simulink model "CombinedTractionLaunchControl"  (R2019b)
settings: Solver=ode1  StartTime=0.0  StopTime=inf  FixedStep=0.0002  RelTol=1e-3
PreLoadFcn:
  | vehicle = 'Car'; if ~length(which('cmself')), cmenv; end
  | CombinedTractionLaunchControl_bus
InitFcn:
  | vehicle = 'Car'; if ~length(which('cmself')), cmenv; end
  | CombinedTractionLaunchControl_bus
libraries: CarMaker4SL x32
(part 2 of 2)

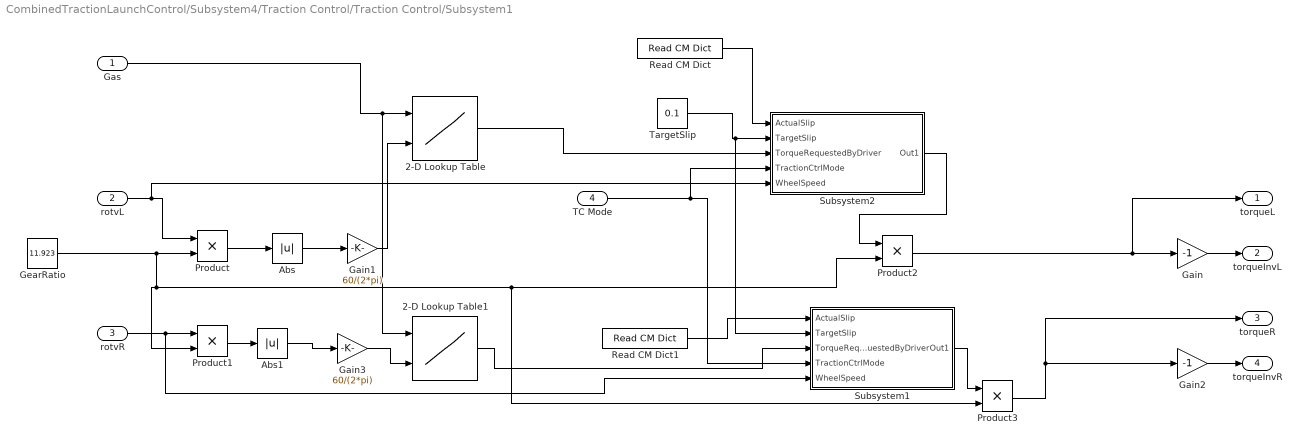
== system CombinedTractionLaunchControl/Subsystem4/Traction Control/Traction Control/Subsystem1 ==
  Gas : Inport
  rotvL : Inport  Port=2
  rotvR : Inport  Port=3
  TC Mode : Inport  Port=4
  2-D Lookup Table : Lookup_n-D  BreakpointsForDimension1=[0 0.2 0.4 0.6 0.8 1]  BreakpointsForDimension2=[0 2000 4000 6000 8000 10000 12000 14000 15000 16000 17000 18000 20000 22000]  Table=[0 0 0 0 0 0 0 0 0 0 0 0 0 0;4 4 4 4 4 4 4 4 4 4 4 4 3 0;8 8 8 8 8 8 8 8 8 8 8 8 6 0;13 13 13 13 13 13 13 13 13 12 12 11 9 0;17 17 17 17 17 17 17 17 17 16 16 15 12 0;21 21 21 21 21 21 21 21 21 20 20 19 15 0]  InternalRulePriority=Speed  RndMeth=Simplest  InputSameDT=on
  2-D Lookup Table1 : Lookup_n-D  BreakpointsForDimension1=[0 0.2 0.4 0.6 0.8 1]  BreakpointsForDimension2=[0 2000 4000 6000 8000 10000 12000 14000 15000 16000 17000 18000 20000 22000]  Table=[0 0 0 0 0 0 0 0 0 0 0 0 0 0;4 4 4 4 4 4 4 4 4 4 4 4 3 0;8 8 8 8 8 8 8 8 8 8 8 8 6 0;13 13 13 13 13 13 13 13 13 12 12 11 9 0;17 17 17 17 17 17 17 17 17 16 16 15 12 0;21 21 21 21 21 21 21 21 21 20 20 19 15 0]  InternalRulePriority=Speed  RndMeth=Simplest  InputSameDT=on
  Abs : Abs
  Abs1 : Abs
  Gain : Gain  Gain=-1
  Gain1 : Gain  Gain=60/(2*pi)
  Gain2 : Gain  Gain=-1
  Gain3 : Gain  Gain=60/(2*pi)
  GearRatio : Constant  Value=11.923
  Product{,1..3} (4 alike) : Product
  Read CM Dict : CarMaker4SL/Read CM Dict  xname=Car.LongSlipFL  xsync=off
  Read CM Dict1 : CarMaker4SL/Read CM Dict  xname=Car.LongSlipFR  xsync=off
  Subsystem1 : Subsystem
  Subsystem2 : Subsystem
  TargetSlip : Constant  Value=0.1
  torqueL : Outport
  torqueInvL : Outport  Port=2
  torqueR : Outport  Port=3
  torqueInvR : Outport  Port=4
  wires:
  Gain/1 -> torqueInvL/1
  Product/1 -> Abs/1
  Gas/1 -> 2-D Lookup Table1/1, 2-D Lookup Table/1
  GearRatio/1 -> Product1/2, Product2/2, Product3/2, Product/2
  rotvL/1 -> Subsystem2/5(WheelSpeed), Product/1
  Product2/1 -> Gain/1, torqueL/1
  Abs/1 -> Gain1/1
  Gain1/1 -> 2-D Lookup Table/2
  Gain2/1 -> torqueInvR/1
  rotvR/1 -> Subsystem1/5(WheelSpeed), Product1/1
  Gain3/1 -> 2-D Lookup Table1/2
  Product1/1 -> Abs1/1
  Abs1/1 -> Gain3/1
  Product3/1 -> torqueR/1, Gain2/1
  Subsystem2/1(Out1) -> Product2/1
  Subsystem1/1(Out1) -> Product3/1
  2-D Lookup Table1/1 -> Subsystem1/3(TorqueRequestedByDriver)
  2-D Lookup Table/1 -> Subsystem2/3(TorqueRequestedByDriver)
  TC Mode/1 -> Subsystem1/4(TractionCtrlMode), Subsystem2/4(TractionCtrlMode)
  TargetSlip/1 -> Subsystem1/2(TargetSlip), Subsystem2/2(TargetSlip)
  Read CM Dict1/1 -> Subsystem1/1(ActualSlip)
  Read CM Dict/1 -> Subsystem2/1(ActualSlip)

== system CombinedTractionLaunchControl/Subsystem4/Launch Control/LaunchControl/Subsystem/If Action Subsystem ==
  In1 : Inport
  Action Port : ActionPort  ActionPortLabel=if(u2< u1)
  Out1 : Outport
  wires:
  In1/1 -> Out1/1

== system CombinedTractionLaunchControl/Subsystem4/Launch Control/LaunchControl/Subsystem/If Action Subsystem1 ==
  In1 : Inport
  Action Port : ActionPort  ActionPortLabel=else
  Out1 : Outport
  wires:
  In1/1 -> Out1/1

== system CombinedTractionLaunchControl/Subsystem4/Launch Control/LaunchControl/Subsystem1/If Action Subsystem ==
  In1 : Inport
  Action Port : ActionPort  ActionPortLabel=if(u2< u1)
  Out1 : Outport
  wires:
  In1/1 -> Out1/1

== system CombinedTractionLaunchControl/Subsystem4/Launch Control/LaunchControl/Subsystem1/If Action Subsystem1 ==
  In1 : Inport
  Action Port : ActionPort  ActionPortLabel=else
  Out1 : Outport
  wires:
  In1/1 -> Out1/1

== system CombinedTractionLaunchControl/Subsystem4/Launch Control/LaunchControl/Subsystem2/If Action Subsystem ==
  In1 : Inport
  Action Port : ActionPort  ActionPortLabel=if(u2< u1)
  Out1 : Outport
  wires:
  In1/1 -> Out1/1

== system CombinedTractionLaunchControl/Subsystem4/Launch Control/LaunchControl/Subsystem2/If Action Subsystem1 ==
  In1 : Inport
  Action Port : ActionPort  ActionPortLabel=else
  Out1 : Outport
  wires:
  In1/1 -> Out1/1

== system CombinedTractionLaunchControl/Subsystem4/Launch Control/LaunchControl/Subsystem3/If Action Subsystem ==
  In1 : Inport
  Action Port : ActionPort  ActionPortLabel=if(u2< u1)
  Out1 : Outport
  wires:
  In1/1 -> Out1/1

== system CombinedTractionLaunchControl/Subsystem4/Launch Control/LaunchControl/Subsystem3/If Action Subsystem1 ==
  In1 : Inport
  Action Port : ActionPort  ActionPortLabel=else
  Out1 : Outport
  wires:
  In1/1 -> Out1/1

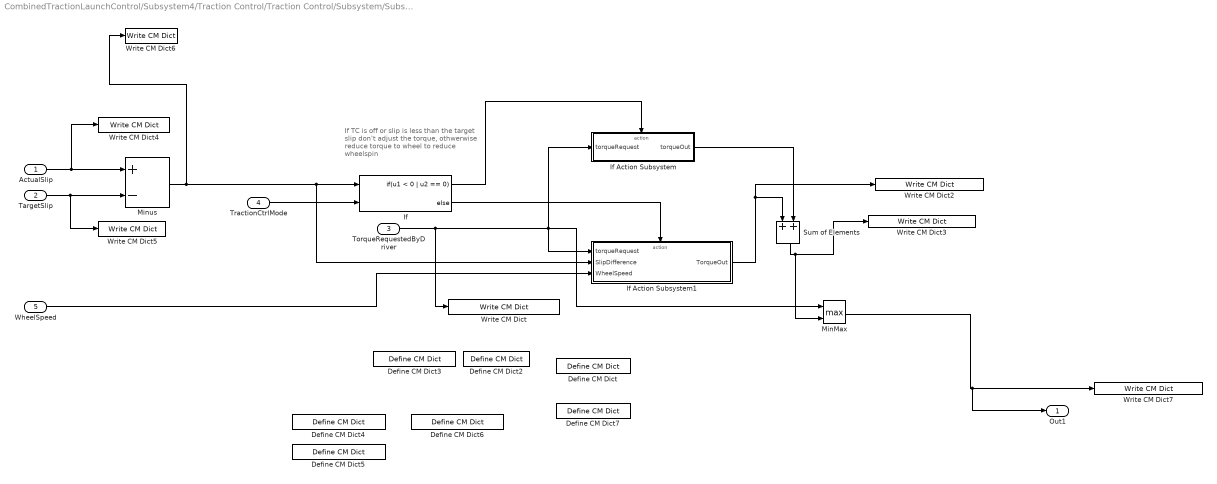
== system CombinedTractionLaunchControl/Subsystem4/Traction Control/Traction Control/Subsystem/Subsystem ==
  note: If TC is off or slip is less than the target slip don't adjust the torque,
      | othwerwise reduce torque to wheel to reduce wheelspin
  ActualSlip : Inport
  TargetSlip : Inport  Port=2
  TorqueRequestedByDriver : Inport  Port=3
  TractionCtrlMode : Inport  Port=4
  WheelSpeed : Inport  Port=5
  Define CM Dict : CarMaker4SL/Define CM Dict  xname=Caleb.TorquePidOut  xmono=off  xtype=Double4  xdvaplace=None  xnstates=0  xfirststate=0  xinitial=0
  Define CM Dict2 : CarMaker4SL/Define CM Dict  xname=Caleb.IfOutput  xmono=off  xtype=Double4  xdvaplace=None  xnstates=0  xfirststate=0  xinitial=0
  Define CM Dict3 : CarMaker4SL/Define CM Dict  xname=Caleb.TorqueRequest  xmono=off  xtype=Double4  xdvaplace=None  xnstates=0  xfirststate=0  xinitial=0
  Define CM Dict4 : CarMaker4SL/Define CM Dict  xname=Caleb.TargetSlip  xmono=off  xtype=Double4  xdvaplace=None  xnstates=0  xfirststate=0  xinitial=0
  Define CM Dict5 : CarMaker4SL/Define CM Dict  xname=Caleb.ActualSlip  xmono=off  xtype=Double4  xdvaplace=None  xnstates=0  xfirststate=0  xinitial=0
  Define CM Dict6 : CarMaker4SL/Define CM Dict  xname=Caleb.DiffSlip  xmono=off  xtype=Double4  xdvaplace=None  xnstates=0  xfirststate=0  xinitial=0
  Define CM Dict7 : CarMaker4SL/Define CM Dict  xname=Caleb.TorqueOut  xmono=off  xtype=Double4  xdvaplace=None  xnstates=0  xfirststate=0  xinitial=0
  If : If  NumInputs=2  IfExpression=u1 < 0 | u2 == 0
  If Action Subsystem : Subsystem  TreatAsAtomicUnit=on
  If Action Subsystem1 : Subsystem  TreatAsAtomicUnit=on
  MinMax : MinMax  Function=max  Inputs=2
  Minus : Sum  Inputs=+-
  Sum of Elements : Sum  Inputs=2
  Write CM Dict : CarMaker4SL/Write CM Dict  xname=Caleb.TorqueRequest  xsync=off
  Write CM Dict2 : CarMaker4SL/Write CM Dict  xname=Caleb.IfOutput  xsync=off
  Write CM Dict3 : CarMaker4SL/Write CM Dict  xname=Caleb.TorquePidOut  xsync=off
  Write CM Dict4 : CarMaker4SL/Write CM Dict  xname=Caleb.TargetSlip  xsync=off
  Write CM Dict5 : CarMaker4SL/Write CM Dict  xname=Caleb.ActualSlip  xsync=off
  Write CM Dict6 : CarMaker4SL/Write CM Dict  xname=Caleb.DiffSlip  xsync=off
  Write CM Dict7 : CarMaker4SL/Write CM Dict  xname=Caleb.TorqueOut  xsync=off
  Out1 : Outport
  wires:
  If Action Subsystem1/1(TorqueOut) -> Write CM Dict2/1, Sum of Elements/1
  TorqueRequestedByDriver/1 -> Write CM Dict/1, If Action Subsystem1/1(torqueRequest), MinMax/1, If Action Subsystem/1(torqueRequest)
  If/1 -> If Action Subsystem/Action
  If Action Subsystem/1(torqueOut) -> Sum of Elements/2
  ActualSlip/1 -> Write CM Dict4/1, Minus/1
  Minus/1 -> Write CM Dict6/1, If Action Subsystem1/2(SlipDifference), If/1
  Sum of Elements/1 -> MinMax/2, Write CM Dict3/1
  TargetSlip/1 -> Write CM Dict5/1, Minus/2
  If/2 -> If Action Subsystem1/Action
  TractionCtrlMode/1 -> If/2
  MinMax/1 -> Out1/1, Write CM Dict7/1
  WheelSpeed/1 -> If Action Subsystem1/3(WheelSpeed)

== system CombinedTractionLaunchControl/Subsystem4/Traction Control/Traction Control/Subsystem/Subsystem1 ==
  note: If TC is off or slip is less than the target slip don't adjust the torque,
      | othwerwise reduce torque to wheel to reduce wheelspin
  ActualSlip : Inport
  TargetSlip : Inport  Port=2
  TorqueRequestedByDriver : Inport  Port=3
  TractionCtrlMode : Inport  Port=4
  WheelSpeed : Inport  Port=5
  If : If  NumInputs=2  IfExpression=u1 < 0 | u2 == 0
  If Action Subsystem : Subsystem  TreatAsAtomicUnit=on
  If Action Subsystem1 : Subsystem  TreatAsAtomicUnit=on
  MinMax : MinMax  Function=max  Inputs=2
  Minus : Sum  Inputs=+-
  Sum of Elements : Sum  Inputs=2
  Out1 : Outport
  wires:
  If Action Subsystem1/1(TorqueOut) -> Sum of Elements/1
  TorqueRequestedByDriver/1 -> If Action Subsystem1/1(torqueRequest), MinMax/1, If Action Subsystem/1(torqueRequest)
  If/1 -> If Action Subsystem/Action
  If Action Subsystem/1(torqueOut) -> Sum of Elements/2
  ActualSlip/1 -> Minus/1
  Minus/1 -> If Action Subsystem1/2(SlipDifference), If/1
  Sum of Elements/1 -> MinMax/2
  TargetSlip/1 -> Minus/2
  If/2 -> If Action Subsystem1/Action
  TractionCtrlMode/1 -> If/2
  MinMax/1 -> Out1/1
  WheelSpeed/1 -> If Action Subsystem1/3(WheelSpeed)

== system CombinedTractionLaunchControl/Subsystem4/Traction Control/Traction Control/Subsystem1/Subsystem1 ==
  note: If TC is off or slip is less than the target slip don't adjust the torque,
      | othwerwise reduce torque to wheel to reduce wheelspin
  ActualSlip : Inport
  TargetSlip : Inport  Port=2
  TorqueRequestedByDriver : Inport  Port=3
  TractionCtrlMode : Inport  Port=4
  WheelSpeed : Inport  Port=5
  If : If  NumInputs=2  IfExpression=u1 < 0 | u2 == 0
  If Action Subsystem : Subsystem  TreatAsAtomicUnit=on
  If Action Subsystem1 : Subsystem  TreatAsAtomicUnit=on
  MinMax : MinMax  Function=max  Inputs=2
  Minus : Sum  Inputs=+-
  Sum of Elements : Sum  Inputs=2
  Out1 : Outport
  wires:
  If Action Subsystem1/1(TorqueOut) -> Sum of Elements/1
  TorqueRequestedByDriver/1 -> If Action Subsystem1/1(torqueRequest), MinMax/1, If Action Subsystem/1(torqueRequest)
  If/1 -> If Action Subsystem/Action
  If Action Subsystem/1(torqueOut) -> Sum of Elements/2
  ActualSlip/1 -> Minus/1
  Minus/1 -> If Action Subsystem1/2(SlipDifference), If/1
  Sum of Elements/1 -> MinMax/2
  TargetSlip/1 -> Minus/2
  If/2 -> If Action Subsystem1/Action
  TractionCtrlMode/1 -> If/2
  MinMax/1 -> Out1/1
  WheelSpeed/1 -> If Action Subsystem1/3(WheelSpeed)

== system CombinedTractionLaunchControl/Subsystem4/Traction Control/Traction Control/Subsystem1/Subsystem2 ==
  note: If TC is off or slip is less than the target slip don't adjust the torque,
      | othwerwise reduce torque to wheel to reduce wheelspin
  ActualSlip : Inport
  TargetSlip : Inport  Port=2
  TorqueRequestedByDriver : Inport  Port=3
  TractionCtrlMode : Inport  Port=4
  WheelSpeed : Inport  Port=5
  If : If  NumInputs=2  IfExpression=u1 < 0 | u2 == 0
  If Action Subsystem : Subsystem  TreatAsAtomicUnit=on
  If Action Subsystem1 : Subsystem  TreatAsAtomicUnit=on
  MinMax : MinMax  Function=max  Inputs=2
  Minus : Sum  Inputs=+-
  Sum of Elements : Sum  Inputs=2
  Out1 : Outport
  wires:
  If Action Subsystem1/1(TorqueOut) -> Sum of Elements/1
  TorqueRequestedByDriver/1 -> MinMax/1, If Action Subsystem1/1(torqueRequest), If Action Subsystem/1(torqueRequest)
  If/1 -> If Action Subsystem/Action
  If Action Subsystem/1(torqueOut) -> Sum of Elements/2
  ActualSlip/1 -> Minus/1
  Minus/1 -> If Action Subsystem1/2(SlipDifference), If/1
  Sum of Elements/1 -> MinMax/2
  TargetSlip/1 -> Minus/2
  If/2 -> If Action Subsystem1/Action
  TractionCtrlMode/1 -> If/2
  MinMax/1 -> Out1/1
  WheelSpeed/1 -> If Action Subsystem1/3(WheelSpeed)

== system CombinedTractionLaunchControl/Subsystem4/Traction Control/Traction Control/Subsystem/Subsystem/If Action Subsystem ==
  torqueRequest : Inport
  Action Port : ActionPort  ActionPortLabel=if(u1 < 0 | u2 == 0)
  torqueOut : Outport
  wires:
  torqueRequest/1 -> torqueOut/1

== system CombinedTractionLaunchControl/Subsystem4/Traction Control/Traction Control/Subsystem/Subsystem/If Action Subsystem1 ==
  torqueRequest : Inport
  SlipDifference : Inport  Port=2
  WheelSpeed : Inport  Port=3
  Action Port : ActionPort  ActionPortLabel=else
  2-D Lookup Table : Lookup_n-D  BreakpointsForDimension1=[0 0.05 0.1 0.15 0.5 2.5]  BreakpointsForDimension2=[0 500 1000 1500 2000]  Table=[0 0 0 0 0;2 2 2 2 2; 5 5 5 5 5; 7 7 7 7 7; 12 12 12 12 12; 50 50 50 50 50]  InternalRulePriority=Speed  RndMeth=Simplest  InputSameDT=on
  Constant : Constant
  Gain : Gain  Gain=1/100
  If : If  IfExpression=u1 > 1
  If Action Subsystem : Subsystem  TreatAsAtomicUnit=on
  If Action Subsystem1 : Subsystem  TreatAsAtomicUnit=on
  Mult : Product  Inputs=**
  Subtract : Sum  Inputs=+-
  Subtract1 : Sum
  TorqueOut : Outport
  wires:
  torqueRequest/1 -> Mult/1
  Mult/1 -> TorqueOut/1
  SlipDifference/1 -> 2-D Lookup Table/1
  WheelSpeed/1 -> 2-D Lookup Table/2
  Constant/1 -> If Action Subsystem/1(torqueRequest), Subtract/1
  Subtract/1 -> Mult/2
  If/2 -> If Action Subsystem1/Action
  If/1 -> If Action Subsystem/Action
  If Action Subsystem/1(torqueOut) -> Subtract1/1
  If Action Subsystem1/1(torqueOut) -> Subtract1/2
  Subtract1/1 -> Subtract/2
  Gain/1 -> If/1, If Action Subsystem1/1(torqueRequest)
  2-D Lookup Table/1 -> Gain/1

== system CombinedTractionLaunchControl/Subsystem4/Traction Control/Traction Control/Subsystem/Subsystem1/If Action Subsystem ==
  torqueRequest : Inport
  Action Port : ActionPort  ActionPortLabel=if(u1 < 0 | u2 == 0)
  torqueOut : Outport
  wires:
  torqueRequest/1 -> torqueOut/1

== system CombinedTractionLaunchControl/Subsystem4/Traction Control/Traction Control/Subsystem/Subsystem1/If Action Subsystem1 ==
  torqueRequest : Inport
  SlipDifference : Inport  Port=2
  WheelSpeed : Inport  Port=3
  Action Port : ActionPort  ActionPortLabel=else
  2-D Lookup Table : Lookup_n-D  BreakpointsForDimension1=[0 0.05 0.1 0.15 0.5 2.5]  BreakpointsForDimension2=[0 500 1000 1500 2000]  Table=[0 0 0 0 0;2 2 2 2 2; 5 5 5 5 5; 7 7 7 7 7; 12 12 12 12 12; 50 50 50 50 50]  InternalRulePriority=Speed  RndMeth=Simplest  InputSameDT=on
  Constant : Constant
  Gain : Gain  Gain=1/100
  If : If  IfExpression=u1 > 1
  If Action Subsystem : Subsystem  TreatAsAtomicUnit=on
  If Action Subsystem1 : Subsystem  TreatAsAtomicUnit=on
  Mult : Product  Inputs=**
  Subtract : Sum  Inputs=+-
  Subtract1 : Sum
  TorqueOut : Outport
  wires:
  torqueRequest/1 -> Mult/1
  Mult/1 -> TorqueOut/1
  SlipDifference/1 -> 2-D Lookup Table/1
  WheelSpeed/1 -> 2-D Lookup Table/2
  Constant/1 -> If Action Subsystem/1(torqueRequest), Subtract/1
  Subtract/1 -> Mult/2
  If/2 -> If Action Subsystem1/Action
  If/1 -> If Action Subsystem/Action
  If Action Subsystem/1(torqueOut) -> Subtract1/1
  If Action Subsystem1/1(torqueOut) -> Subtract1/2
  Subtract1/1 -> Subtract/2
  Gain/1 -> If/1, If Action Subsystem1/1(torqueRequest)
  2-D Lookup Table/1 -> Gain/1

== system CombinedTractionLaunchControl/Subsystem4/Traction Control/Traction Control/Subsystem1/Subsystem1/If Action Subsystem ==
  torqueRequest : Inport
  Action Port : ActionPort  ActionPortLabel=if(u1 < 0 | u2 == 0)
  torqueOut : Outport
  wires:
  torqueRequest/1 -> torqueOut/1

== system CombinedTractionLaunchControl/Subsystem4/Traction Control/Traction Control/Subsystem1/Subsystem1/If Action Subsystem1 ==
  torqueRequest : Inport
  SlipDifference : Inport  Port=2
  WheelSpeed : Inport  Port=3
  Action Port : ActionPort  ActionPortLabel=else
  2-D Lookup Table : Lookup_n-D  BreakpointsForDimension1=[0 0.05 0.1 0.15 0.5 2.5]  BreakpointsForDimension2=[0 500 1000 1500 2000]  Table=[0 0 0 0 0;2 2 2 2 2; 5 5 5 5 5; 7 7 7 7 7; 12 12 12 12 12; 50 50 50 50 50]  InternalRulePriority=Speed  RndMeth=Simplest  InputSameDT=on
  Constant : Constant
  Gain : Gain  Gain=1/100
  If : If  IfExpression=u1 > 1
  If Action Subsystem : Subsystem  TreatAsAtomicUnit=on
  If Action Subsystem1 : Subsystem  TreatAsAtomicUnit=on
  Mult : Product  Inputs=**
  Subtract : Sum  Inputs=+-
  Subtract1 : Sum
  TorqueOut : Outport
  wires:
  torqueRequest/1 -> Mult/1
  Mult/1 -> TorqueOut/1
  SlipDifference/1 -> 2-D Lookup Table/1
  WheelSpeed/1 -> 2-D Lookup Table/2
  Constant/1 -> If Action Subsystem/1(torqueRequest), Subtract/1
  Subtract/1 -> Mult/2
  If/2 -> If Action Subsystem1/Action
  If/1 -> If Action Subsystem/Action
  If Action Subsystem/1(torqueOut) -> Subtract1/1
  If Action Subsystem1/1(torqueOut) -> Subtract1/2
  Subtract1/1 -> Subtract/2
  Gain/1 -> If/1, If Action Subsystem1/1(torqueRequest)
  2-D Lookup Table/1 -> Gain/1

== system CombinedTractionLaunchControl/Subsystem4/Traction Control/Traction Control/Subsystem1/Subsystem2/If Action Subsystem ==
  torqueRequest : Inport
  Action Port : ActionPort  ActionPortLabel=if(u1 < 0 | u2 == 0)
  torqueOut : Outport
  wires:
  torqueRequest/1 -> torqueOut/1

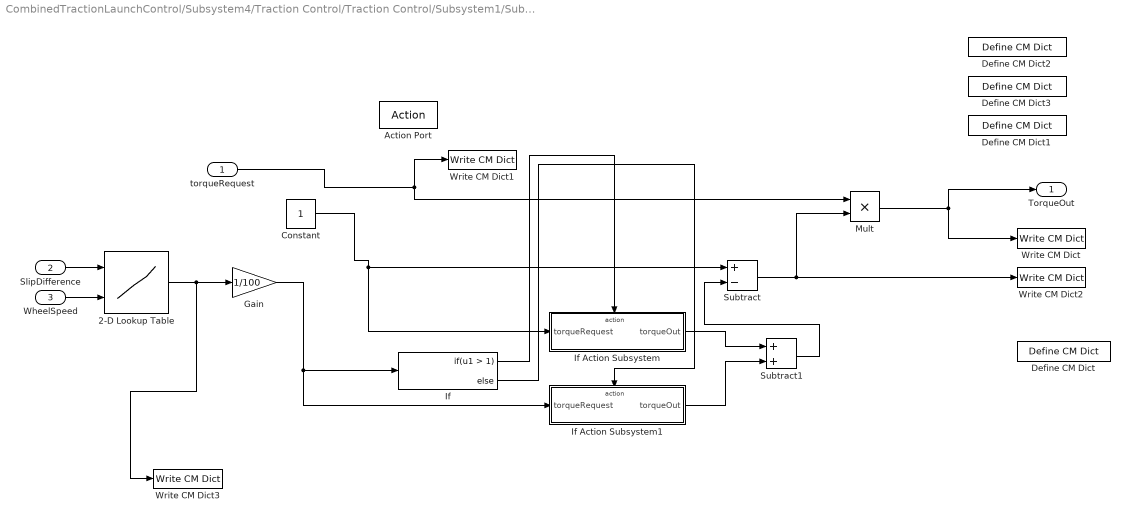
== system CombinedTractionLaunchControl/Subsystem4/Traction Control/Traction Control/Subsystem1/Subsystem2/If Action Subsystem1 ==
  torqueRequest : Inport
  SlipDifference : Inport  Port=2
  WheelSpeed : Inport  Port=3
  Action Port : ActionPort  ActionPortLabel=else
  2-D Lookup Table : Lookup_n-D  BreakpointsForDimension1=[0 0.05 0.1 0.15 0.5 2.5]  BreakpointsForDimension2=[0 500 1000 1500 2000]  Table=[0 0 0 0 0;2 2 2 2 2; 5 5 5 5 5; 7 7 7 7 7; 12 12 12 12 12; 50 50 50 50 50]  InternalRulePriority=Speed  RndMeth=Simplest  InputSameDT=on
  Constant : Constant
  Define CM Dict : CarMaker4SL/Define CM Dict  xname=Caleb.torqueOld  xmono=off  xtype=Double4  xdvaplace=None  xnstates=0  xfirststate=0  xinitial=0
  Define CM Dict1 : CarMaker4SL/Define CM Dict  xname=Caleb.torqueNew  xmono=off  xtype=Double4  xdvaplace=None  xnstates=0  xfirststate=0  xinitial=0
  Define CM Dict2 : CarMaker4SL/Define CM Dict  xname=Caleb.Percent  xmono=off  xtype=Double4  xdvaplace=None  xnstates=0  xfirststate=0  xinitial=0
  Define CM Dict3 : CarMaker4SL/Define CM Dict  xname=Caleb.Table  xmono=off  xtype=Double4  xdvaplace=None  xnstates=0  xfirststate=0  xinitial=0
  Gain : Gain  Gain=1/100
  If : If  IfExpression=u1 > 1
  If Action Subsystem : Subsystem  TreatAsAtomicUnit=on
  If Action Subsystem1 : Subsystem  TreatAsAtomicUnit=on
  Mult : Product  Inputs=**
  Subtract : Sum  Inputs=+-
  Subtract1 : Sum
  Write CM Dict : CarMaker4SL/Write CM Dict  xname=Caleb.torqueNew  xsync=off
  Write CM Dict1 : CarMaker4SL/Write CM Dict  xname=Caleb.torqueOld  xsync=off
  Write CM Dict2 : CarMaker4SL/Write CM Dict  xname=Caleb.Percent  xsync=off
  Write CM Dict3 : CarMaker4SL/Write CM Dict  xname=Caleb.Table  xsync=off
  TorqueOut : Outport
  wires:
  torqueRequest/1 -> Write CM Dict1/1, Mult/1
  Mult/1 -> Write CM Dict/1, TorqueOut/1
  SlipDifference/1 -> 2-D Lookup Table/1
  WheelSpeed/1 -> 2-D Lookup Table/2
  Constant/1 -> If Action Subsystem/1(torqueRequest), Subtract/1
  Subtract/1 -> Write CM Dict2/1, Mult/2
  If/2 -> If Action Subsystem1/Action
  If/1 -> If Action Subsystem/Action
  If Action Subsystem/1(torqueOut) -> Subtract1/1
  If Action Subsystem1/1(torqueOut) -> Subtract1/2
  Subtract1/1 -> Subtract/2
  Gain/1 -> If/1, If Action Subsystem1/1(torqueRequest)
  2-D Lookup Table/1 -> Write CM Dict3/1, Gain/1

== system CombinedTractionLaunchControl/Subsystem4/Traction Control/Traction Control/Subsystem/Subsystem/If Action Subsystem1/If Action Subsystem ==
  torqueRequest : Inport
  Action Port : ActionPort  ActionPortLabel=if(u1 > 1)
  torqueOut : Outport
  wires:
  torqueRequest/1 -> torqueOut/1

== system CombinedTractionLaunchControl/Subsystem4/Traction Control/Traction Control/Subsystem/Subsystem/If Action Subsystem1/If Action Subsystem1 ==
  torqueRequest : Inport
  Action Port : ActionPort  ActionPortLabel=else
  torqueOut : Outport
  wires:
  torqueRequest/1 -> torqueOut/1

== system CombinedTractionLaunchControl/Subsystem4/Traction Control/Traction Control/Subsystem/Subsystem1/If Action Subsystem1/If Action Subsystem ==
  torqueRequest : Inport
  Action Port : ActionPort  ActionPortLabel=if(u1 > 1)
  torqueOut : Outport
  wires:
  torqueRequest/1 -> torqueOut/1

== system CombinedTractionLaunchControl/Subsystem4/Traction Control/Traction Control/Subsystem/Subsystem1/If Action Subsystem1/If Action Subsystem1 ==
  torqueRequest : Inport
  Action Port : ActionPort  ActionPortLabel=else
  torqueOut : Outport
  wires:
  torqueRequest/1 -> torqueOut/1

== system CombinedTractionLaunchControl/Subsystem4/Traction Control/Traction Control/Subsystem1/Subsystem1/If Action Subsystem1/If Action Subsystem ==
  torqueRequest : Inport
  Action Port : ActionPort  ActionPortLabel=if(u1 > 1)
  torqueOut : Outport
  wires:
  torqueRequest/1 -> torqueOut/1

== system CombinedTractionLaunchControl/Subsystem4/Traction Control/Traction Control/Subsystem1/Subsystem1/If Action Subsystem1/If Action Subsystem1 ==
  torqueRequest : Inport
  Action Port : ActionPort  ActionPortLabel=else
  torqueOut : Outport
  wires:
  torqueRequest/1 -> torqueOut/1

== system CombinedTractionLaunchControl/Subsystem4/Traction Control/Traction Control/Subsystem1/Subsystem2/If Action Subsystem1/If Action Subsystem ==
  torqueRequest : Inport
  Action Port : ActionPort  ActionPortLabel=if(u1 > 1)
  torqueOut : Outport
  wires:
  torqueRequest/1 -> torqueOut/1

== system CombinedTractionLaunchControl/Subsystem4/Traction Control/Traction Control/Subsystem1/Subsystem2/If Action Subsystem1/If Action Subsystem1 ==
  torqueRequest : Inport
  Action Port : ActionPort  ActionPortLabel=else
  torqueOut : Outport
  wires:
  torqueRequest/1 -> torqueOut/1
